simulink model "ComControl"  (R2020a)
settings: Solver=ode3  StartTime=0.0  StopTime=10.0  RelTol=1e-3
PreLoadFcn:
  | % Lidar parameters
  | 
  | scanAngles = linspace(-pi/2,pi/2,360);
  | scanMaxRange = 3.5;
  | scanSensorOffset = [0,0];
undefined symbols (not defined in the file or in its folder): X, Y
libraries: robotlib x3
settings Model: Creator=Pierre  LastModifiedBy=pierre
settings OptimizationCC: EnhancedBackFolding=on  PassReuseOutputArgsAs=Individual arguments  ZeroExternalMemoryAtStartup=off  ZeroInternalMemoryAtStartup=off  MaxStackSize=64  OptimizeBlockOrder=speed  DifferentSizesBufferReuse=on  OptimizationCustomize=off  EfficientTunableParamExpr=on
settings DebuggingCC: ParameterTunabilityLossMsg=error
settings HardwareCC: ProdBitPerPointer=32  ProdBitPerSizeT=32  ProdBitPerPtrDiffT=32  ProdLargestAtomicFloat=None  ProdIntDivRoundTo=Undefined  ProdEndianess=Unspecified  ProdWordSize=32  ProdHWDeviceType=Generic->Unspecified (assume 32-bit Generic)
settings SFSimCC: MATLABDynamicMemAlloc=off
settings RTWCC: SystemTargetFile=ert.tlc  HardwareBoard=Robot Operating System (ROS)  TemplateMakefile=ert_default_tmf  Toolchain=Catkin  TargetLang=C++
settings CodeAppCC: ForceParamTrailComments=on  IgnoreCustomStorageClasses=off  OperatorAnnotations=on  SimulinkDataObjDesc=on  SFDataObjDesc=on  InsertBlockDesc=on
settings ERTTargetCC: SupportVariableSizeSignals=on

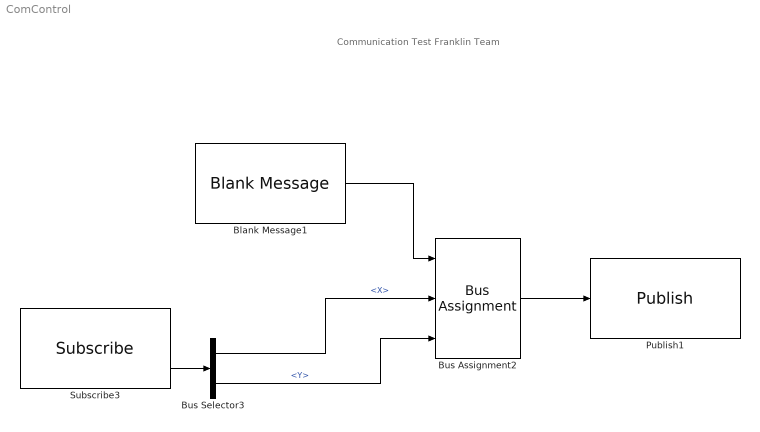
== system ComControl ==
  note: Communication Test
      |
      | Franklin Team
  Blank Message1 : robotlib/Blank Message  messageClass=Message  entityType=geometry_msgs/Pose2D  messageType=geometry_msgs/Pose2D  SampleTime=inf
  Bus Assignment2 : BusAssignment  AssignedSignals=X,Y
  Bus Selector3 : BusSelector  OutputSignals=X,Y
  Publish1 : robotlib/Publish  topicSource=Specify your own  topic=/test  messageType=geometry_msgs/Pose2D  messageQueueLength=1
  Subscribe3 : robotlib/Subscribe  topicSource=Specify your own  topic=/destination  messageType=geometry_msgs/Pose2D  sampleTime=1  messageQueueLength=1
  wires:
  Bus Selector3/1 -> Bus Assignment2/2  "<X>"
  Bus Selector3/2 -> Bus Assignment2/3  "<Y>"
  Blank Message1/1 -> Bus Assignment2/1
  Subscribe3/2 -> Bus Selector3/1
  Bus Assignment2/1 -> Publish1/1
